simulink model "PID"  (R2015b)
settings: Solver=VariableStepAuto  StartTime=0.0  StopTime=10.0  RelTol=1e-3
values from neighbouring files (symbols this model uses):
  L = 4.5    [controller_test.m]    (also in path_follower_main.m)
libraries: simulink x2
settings Model: Creator=Mitch  LastModifiedBy=Mitch

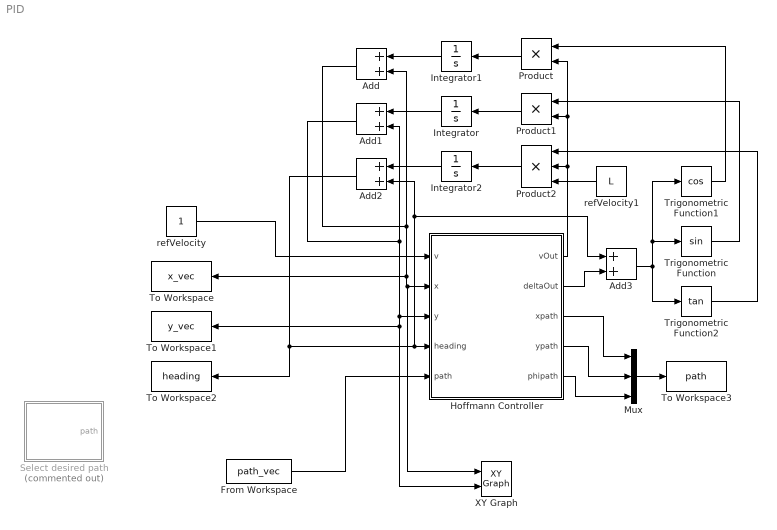
== system PID ==
  Add{,1..3} (4 alike) : Sum
  From Workspace : FromWorkspace  VariableName=path_vec  OutDataTypeStr=double  SampleTime=0  OutputAfterFinalValue=Holding final value
  Hoffmann Controller : Subsystem
  Integrator : Integrator
  Integrator1 : Integrator
  Integrator2 : Integrator
  Mux : Mux  Inputs=3
  Product : Product
  Product1 : Product
  Product2 : Product  Inputs=3
  Select desired path : Subsystem  Commented=on
  To Workspace : ToWorkspace  VariableName=x_vec  SaveFormat=Structure With Time  SampleTime=-1
  To Workspace1 : ToWorkspace  VariableName=y_vec  SaveFormat=Structure With Time  SampleTime=-1
  To Workspace2 : ToWorkspace  VariableName=heading  SaveFormat=Structure With Time  SampleTime=-1
  To Workspace3 : ToWorkspace  VariableName=path  SaveFormat=Structure With Time  SampleTime=-1
  Trigonometric Function : Trigonometry
  Trigonometric Function1 : Trigonometry  Operator=cos
  Trigonometric Function2 : Trigonometry  Operator=tan
  XY Graph : simulink/Sinks/XY Graph  xmin=-50  xmax=50  ymin=-50  ymax=50  st=-1
  refVelocity : Constant
  refVelocity1 : Constant  Value=L
  wires:
  Hoffmann Controller/1(vOut) -> Product2/2, Product/2, Product1/2
  Add/1 -> Add/2, To Workspace/1, XY Graph/1, Hoffmann Controller/2(x)
  Add1/1 -> To Workspace1/1, XY Graph/2, Hoffmann Controller/3(y), Add1/2
  Trigonometric Function1/1 -> Product/1
  Trigonometric Function/1 -> Product1/1
  Integrator1/1 -> Add/1
  Product/1 -> Integrator1/1
  Integrator/1 -> Add1/1
  Product1/1 -> Integrator/1
  refVelocity/1 -> Hoffmann Controller/1(v)
  Trigonometric Function2/1 -> Product2/1
  Product2/1 -> Integrator2/1
  Integrator2/1 -> Add2/1
  Add2/1 -> Add2/2, Add3/1, Hoffmann Controller/4(heading), To Workspace2/1
  Hoffmann Controller/2(deltaOut) -> Add3/2
  Add3/1 -> Trigonometric Function2/1, Trigonometric Function/1, Trigonometric Function1/1
  Hoffmann Controller/4(ypath) -> Mux/2
  Hoffmann Controller/5(phipath) -> Mux/3
  Mux/1 -> To Workspace3/1
  Hoffmann Controller/3(xpath) -> Mux/1
  refVelocity1/1 -> Product2/3
  From Workspace/1 -> Hoffmann Controller/5(path)

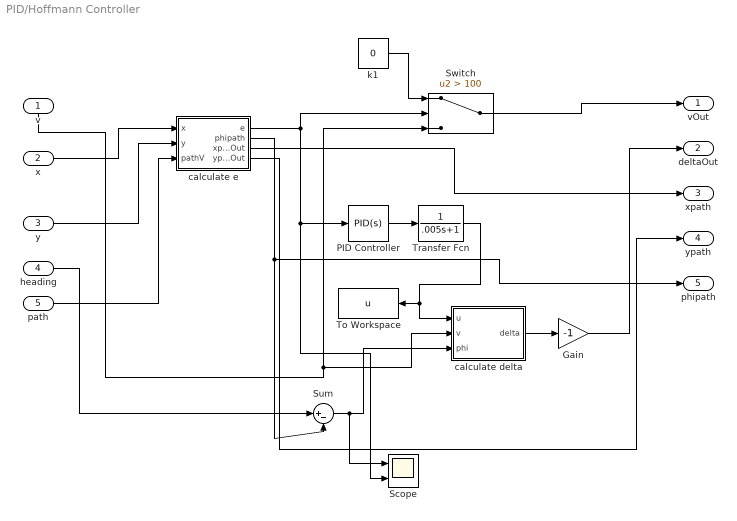
== system PID/Hoffmann Controller ==
  v : Inport
  x : Inport  Port=2
  y : Inport  Port=3
  heading : Inport  Port=4
  path : Inport  Port=5
  Gain : Gain  Gain=-1
  PID Controller : simulink/Continuous/PID Controller  Controller=PID  TimeDomain=Continuous-time  SampleTime=-1  IntegratorMethod=Forward Euler  FilterMethod=Forward Euler  Form=Parallel  UseFilter=on  ControllerParametersSource=internal  P=.1  I=0  D=.1  N=100  InitialConditionSource=internal  InitialConditionForIntegrator=0  InitialConditionForFilter=0  ExternalReset=none  LimitOutput=off  UpperSaturationLimit=inf  LowerSaturationLimit=-inf  LinearizeAsGain=on  AntiWindupMode=none  Kb=1  TrackingMode=off  Kt=1  PParamMin=[]  PParamMax=[]  IParamMin=[]  IParamMax=[]  DParamMin=[]  DParamMax=[]  NParamMin=[]  NParamMax=[]  KbParamMin=[]  KbParamMax=[]  KtParamMin=[]  KtParamMax=[]  POutMin=[]  POutMax=[]  IOutMin=[]  IOutMax=[]  DOutMin=[]  DOutMax=[]  NOutMin=[]  NOutMax=[]  KbOutMin=[]  KbOutMax=[]  KtOutMin=[]  KtOutMax=[]  IntegratorOutMin=[]  IntegratorOutMax=[]  FilterOutMin=[]  FilterOutMax=[]  SumOutMin=[]  SumOutMax=[]  SumI1OutMin=[]  SumI1OutMax=[]  SumI2OutMin=[]  SumI2OutMax=[]  SumI3OutMin=[]  SumI3OutMax=[]  SumDOutMin=[]  SumDOutMax=[]  SaturationOutMin=[]  SaturationOutMax=[]  IntegratorContinuousStateAttributes=''  IntegratorStateMustResolveToSignalObject=off  IntegratorRTWStateStorageClass=Auto  FilterContinuousStateAttributes=''  FilterStateMustResolveToSignalObject=off  FilterRTWStateStorageClass=Auto  DifferentiatorICPrevScaledInput=0  DifferentiatorOutMin=[]  DifferentiatorOutMax=[]
  Scope : Scope  NumInputPorts=2
  Sum : Sum  Inputs=|+-
  Switch : Switch  Criteria=u2 > Threshold  Threshold=100
  To Workspace : ToWorkspace  VariableName=u  SaveFormat=Timeseries  SampleTime=-1
  Transfer Fcn : TransferFcn  Denominator=[.005 1]
  calculate delta : MATLAB Function  TreatAsAtomicUnit=on
  calculate e : MATLAB Function  TreatAsAtomicUnit=on
  k1 : Constant  Value=0
  vOut : Outport
  deltaOut : Outport  Port=2
  xpath : Outport  Port=3
  ypath : Outport  Port=4
  phipath : Outport  Port=5
  wires:
  v/1 -> Switch/3, calculate delta/2(v)
  path/1 -> calculate e/3(pathV)
  x/1 -> calculate e/1(x)
  y/1 -> calculate e/2(y)
  calculate e/2(phipath) -> phipath/1, Sum/2
  calculate e/1(e) -> Switch/2, PID Controller/1, Scope/2
  Sum/1 -> Scope/1, calculate delta/3(phi)
  calculate e/3(xpathOut) -> xpath/1
  calculate e/4(ypathOut) -> ypath/1
  Switch/1 -> vOut/1
  k1/1 -> Switch/1
  heading/1 -> Sum/1
  calculate delta/1(delta) -> Gain/1
  Gain/1 -> deltaOut/1
  PID Controller/1 -> Transfer Fcn/1
  Transfer Fcn/1 -> calculate delta/1(u), To Workspace/1

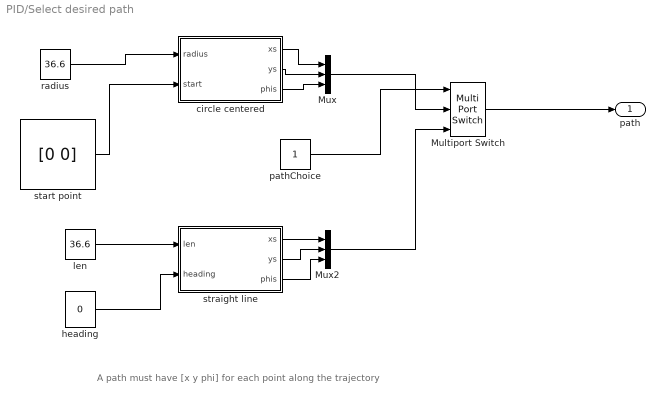
== system PID/Select desired path ==
  note: A path must have [x y phi] for each point along the trajectory
  Multiport Switch : MultiPortSwitch  Inputs=2
  Mux : Mux  Inputs=3
  Mux2 : Mux  Inputs=3
  circle centered : MATLAB Function  TreatAsAtomicUnit=on
  heading : Constant  Value=0
  len : Constant  Value=36.6
  "pathChoice " : Constant
  radius : Constant  Value=36.6
  start point : Constant  Value=[0 0]
  straight line : MATLAB Function  TreatAsAtomicUnit=on
  path : Outport
  wires:
  radius/1 -> circle centered/1(radius)
  start point/1 -> circle centered/2(start)
  "pathChoice "/1 -> Multiport Switch/1
  circle centered/2(ys) -> Mux/2
  circle centered/1(xs) -> Mux/1
  Multiport Switch/1 -> path/1
  len/1 -> straight line/1(len)
  heading/1 -> straight line/2(heading)
  straight line/1(xs) -> Mux2/1
  straight line/2(ys) -> Mux2/2
  Mux2/1 -> Multiport Switch/3
  Mux/1 -> Multiport Switch/2
  straight line/3(phis) -> Mux2/3
  circle centered/3(phis) -> Mux/3

== matlab function PID/Hoffmann Controller/calculate e ==
  data: e output; x input; y input; pathV input; phipath output; xpathOut output; ypathOut output
function [e,phipath,xpathOut,ypathOut] = fcn(x,y,pathV)
%#codegen
path=reshape(pathV,[],3);
x1 = path(1,1);
y1 = path(1,2);
phi1=path(1,3);
etmp = inf;
e = inf;
index=1;
% find the nearest x,y
for i=1:length(path)
   etmp = sqrt((x-path(i,1))^2+(y-path(i,2))^2);
   if( etmp < e ) 
       e = etmp;
       index=i;
   end
end

xpathOut=path(index,1);
ypathOut=path(index,2);
phipath=path(index,3);

ex1 = (path(index,1)-x);
ey1 = (path(index,2)-y);
ex2 = cos(phipath);
ey2 = sin(phipath);
sinnnn = ex1*ey2-ey1*ex2;
e = sign(sinnnn)*e;

== matlab function PID/Hoffmann Controller/calculate delta ==
  data: delta output; u input; v input; phi input
function delta = fcn(u,v,phi)
%#codegen
if( abs(v) < eps )
    v = eps;
end

% if phi is greater than pi (or less than -pi), then 
% we normalize to between [-pi,pi]
if( phi < -pi )
    phi = phi+2*pi;
elseif( phi > pi )
    phi = phi-2*pi;
end

delta = phi + atan2(u,v);

== matlab function PID/Select desired path/circle centered ==
  data: xs output; radius input; start input; ys output; phis output
function [xs,ys,phis] = fcn(radius,start)
%#codegen
angles=linspace(-pi,pi,300);
r = radius*exp(angles*1j);
xs = real(r)-radius+start(1);
ys = imag(r)+start(2);
phis=(pi/2)+angles;

% % % To visualize the angles, run this code:
% radius=3.6; start=[0 0];
% angles=linspace(-pi,pi,10);
% r = radius*exp(angles*1j);
% xs = real(r)-radius+start(1);
% ys = imag(r)+start(2);
% % since the direction of travel is in the 'x' direction, the 
% % heading (phi) matchines the angle of the circle
% phis=(pi/2)+angles;
% xends=.5*cos(phis);yends=.5*sin(phis);
% figure;plot(xs,ys);hold on; quiver(xs,ys,xends,yends);axis equal;hold off

== matlab function PID/Select desired path/straight line ==
  data: xs output; len input; heading input; ys output; phis output
function [xs,ys,phis] = fcn(len,heading)
%#codegen
r = linspace(0,len,300);
xs = r*cos(heading);
ys = r*sin(heading);
phis = heading*ones(1,length(r));
